simulink model "Projeto_Final_versao_1_M24"  (R2024b)
settings: Solver=VariableStepAuto  StartTime=0  StopTime=144  FixedStep=0.1  RelTol=1e-3
model workspace (MAT data in the model file):
  variavelteste = 0
libraries: visiontextngfix x2, spsACVoltageSourceLib x1, spsCurrentMeasurementLib x1, spsSeriesRLCBranchLib x1, spspowerguiLib x1
settings Model: Creator=Henrique  LastModifiedBy=Guilherme Moreira
settings DebuggingCC: UnconnectedInputMsg=warning  UnconnectedOutputMsg=warning  UnconnectedLineMsg=warning
settings ModelReferenceCC: EnableRefExpFcnMdlSchedulingChecks=on
settings RTWCC: GPUComputeCapability=3.5  DLArmComputeVersion=19.05

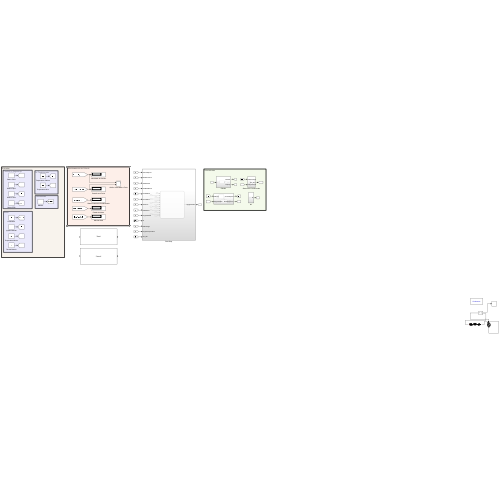
[thumbnail: Simulink's stored preview of the top-level diagram]
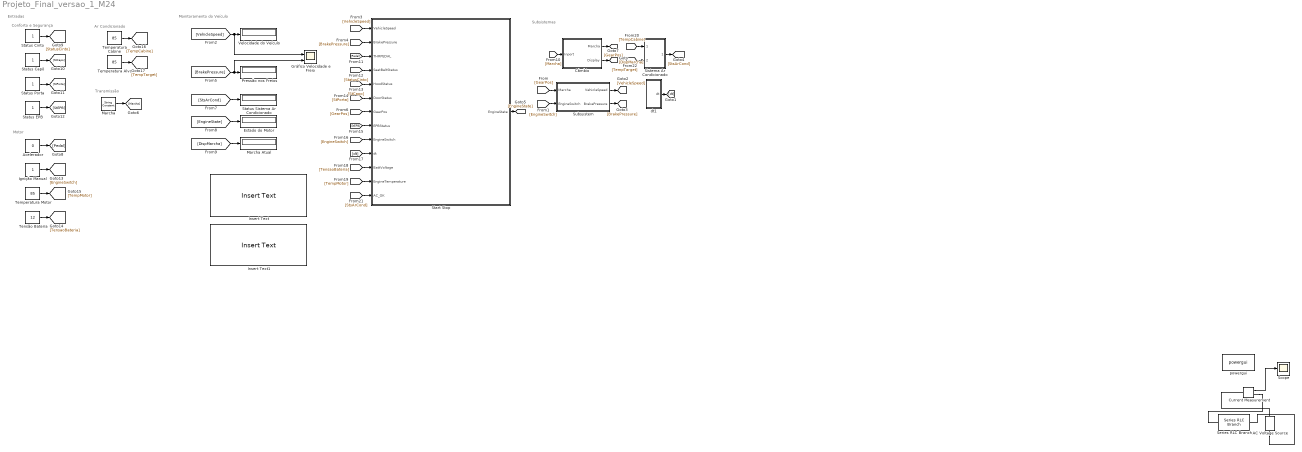
== system Projeto_Final_versao_1_M24 ==
  note: Transmissão
  note: Motor
  note: Conforto e Segurança
  note: Ar Condicionado
  note: Entradas
  note: Subsistemas
  note: Monitoramento do Veículo
  AC Voltage Source : spsACVoltageSourceLib/AC Voltage Source  Amplitude=100  Phase=0  Frequency=60  SampleTime=0  Measurements=None  BusType=swing  Pref=10e3  Qref=0  Qmin=-inf  Qmax=+inf
  Acelerador : Constant  Value=0
  Current Measurement : spsCurrentMeasurementLib/Current Measurement  PhasorSimulation=off  OutputType=Complex  PSBequivalent=0
  Câmbio : Subsystem
  Estado do Motor : Display
  Gráfico Velocidade e Freio : Scope  NumInputPorts=2
  Ignição Manual : Constant
  Insert Text : visiontextngfix/Insert Text  inputType=Obsolete  theText='Teste'  getTextLocFrom=Specify via dialog  textLoc=[1 1]  getTextColorFrom=Specify via dialog  textColor=[0 0 0]  getTextIntensityFrom=Specify via dialog  textIntensity=0  getTextOpacityFrom=Specify via dialog  textOpacity=1.0  dummyVar2=0  dummyVar3=0  dummyVar4=0  imagePorts=One multidimensional signal  isInputTransposed=off  fontFace=LucidaSansRegular  dummyVar1=0  blockFontSize=12  antiAliased=on
  Insert Text1 : visiontextngfix/Insert Text  inputType=Obsolete  theText='Teste2'  getTextLocFrom=Specify via dialog  textLoc=[1 1]  getTextColorFrom=Specify via dialog  textColor=[0 0 0]  getTextIntensityFrom=Specify via dialog  textIntensity=0  getTextOpacityFrom=Specify via dialog  textOpacity=1.0  dummyVar2=0  dummyVar3=0  dummyVar4=0  imagePorts=One multidimensional signal  isInputTransposed=off  fontFace=LucidaSansRegular  dummyVar1=0  blockFontSize=12  antiAliased=on
  Marcha : StringConstant  String="\"D\""
  Marcha Atual : Display
  Pressão nos Freios : Display
  Scope : Scope
  Series RLC Branch : spsSeriesRLCBranchLib/Series RLC Branch  LConnTagsString=__new0  RConnTagsString=__new0  BranchType=RLC  Resistance=1  Inductance=1e-3  SetiL0=off  InitialCurrent=0  Capacitance=1e-6  Setx0=off  InitialVoltage=0  Measurements=None
  Sistema Ar Condicionado : Subsystem
  Start Stop : Subsystem
  Status Capô : Constant
  Status Cinto : Constant
  Status EPB : Constant
  Status Porta : Constant
  Status Sistema Ar Condicionado : Display
  Subsystem : Subsystem
  Temperatura Alvo : Constant  Value=85
  Temperatura Cabine : Constant  Value=85
  Temperatura Motor : Constant  Value=85
  Tensão Bateria : Constant  Value=12
  Velocidade do Veículo : Display
  dt1 : Subsystem
  powergui : spspowerguiLib/powergui  Priority=1  SimulationMode=Continuous  SampleTime=50e-6  frequency=60  Iterations=50  frequencyindice=60  Pbase=100e6  ErrMax=1e-4  UnitsV=kV  UnitsW=MW  buscounter=0  FunctionMessages=off  echomessages=off  EnableUseOfTLC=off  CurrentSourceSwitches=off  DisableSnubberDevices=off  DisableRonSwitches=off  DisableVfSwitches=off  DisplayEquations=off  AutomaticDiscreteSolvers=off  SolverType=Tustin/Backward Euler (TBE)  Interpol=off  ExternalGateDelay=off  methode=off  Ts=100  x0status=blocks  SPID=on  SwTol=0  HookPort=off  NonlinearTolerance=1e-4  nMaxIteration=100  ContinueOnMaxIteration=off  RestoreLinks=warning  ResistiveCurrentMeasurement=off  Frange=[0:2:500]  Ylog=off  Xlog=on  ShowGrid=off  save=off  variable=ZData  structure=0  ZoomFFT=off  StartTime=0.0  cycles=1  DisplayStyle=1  fundamental=60  FreqAxis=off  MaxFrequency=1000  frequencyindicesteady=1  RmsSteady=1  display=off
  wires:
  Current Measurement/1 -> Scope/1
  [dt] -> Start Stop/10(dt)
  Start Stop/1(EngineState) -> [EngineState]
  Sistema Ar Condicionado/1(AC_OK) -> [StsArCond]
  [VehicleSpeed] -> Start Stop/1(VehicleSpeed)
  [BrakePressure] -> Start Stop/2(BrakePressure)
  [VehicleSpeed] -> Gráfico Velocidade e Freio/1, Velocidade do Veículo/1
  [BrakePressure] -> Gráfico Velocidade e Freio/2, Pressão nos Freios/1
  [StsArCond] -> Status Sistema Ar Condicionado/1
  [EngineState] -> Estado do Motor/1
  [DispMarcha] -> Marcha Atual/1
  Marcha/1 -> [Marcha]
  [Marcha] -> Câmbio/1(Inport)
  Câmbio/1(Marcha) -> [GearPos]
  Câmbio/2(Display) -> [DispMarcha]
  [GearPos] -> Start Stop/7(GearPos)
  Acelerador/1 -> [Pedal]
  Status Cinto/1 -> [StatusCinto]
  Status Capô/1 -> [StCapo]
  Status Porta/1 -> [StPorta]
  Status EPB/1 -> [StEPB]
  Ignição Manual/1 -> [EngineSwitch]
  [Pedal] -> Start Stop/3(THRPEDAL)
  [StatusCinto] -> Start Stop/4(SeatBeltStatus)
  [StCapo] -> Start Stop/5(HoodStatus)
  [StPorta] -> Start Stop/6(DoorStatus)
  [StEPB] -> Start Stop/8(EPBStatus)
  [EngineSwitch] -> Start Stop/9(EngineSwitch)
  dt1/1(dt) -> [dt]
  Tensão Bateria/1 -> [TensaoBateria]
  [TensaoBateria] -> Start Stop/11(BattVoltage)
  [TempMotor] -> Start Stop/12(EngineTemperature)
  Temperatura Motor/1 -> [TempMotor]
  [StsArCond] -> Start Stop/13(AC_OK)
  [GearPos] -> Subsystem/1(Marcha)
  [EngineSwitch] -> Subsystem/2(EngineSwitch)
  Subsystem/1(VehicleSpeed) -> [VehicleSpeed]
  Subsystem/2(BrakePressure) -> [BrakePressure]
  Temperatura Alvo/1 -> [TempTarget]
  Temperatura Cabine/1 -> [TempCabine]
  [TempCabine] -> Sistema Ar Condicionado/1(CabinTemperature)
  [TempTarget] -> Sistema Ar Condicionado/2(TargetTemperature)
  connections:
  AC Voltage Source/LConn1 -- Series RLC Branch/RConn1
  AC Voltage Source/RConn1 -- Current Measurement/LConn1
  Current Measurement/RConn1 -- Series RLC Branch/LConn1

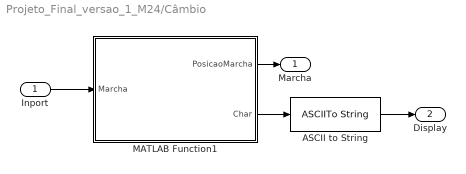
== system Projeto_Final_versao_1_M24/Câmbio ==
  Inport : Inport
  ASCII to String : ASCIIToString
  MATLAB Function1 : MATLAB Function  TreatAsAtomicUnit=on
  Marcha : Outport
  Display : Outport  Port=2
  wires:
  MATLAB Function1/1(PosicaoMarcha) -> Marcha/1
  MATLAB Function1/2(Char) -> ASCII to String/1
  ASCII to String/1 -> Display/1
  Inport/1 -> MATLAB Function1/1(Marcha)

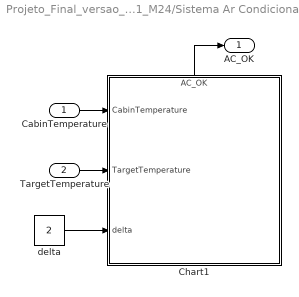
== system Projeto_Final_versao_1_M24/Sistema Ar Condicionado ==
  CabinTemperature : Inport
  TargetTemperature : Inport  Port=2
  Chart1 : Stateflow chart  TreatAsAtomicUnit=on
      settings: PortSchema="{\"entries\":[{\"content\":{\"sides\":[{\"content\":{\"connectorIds\":[\"In1\",\"In2\",\"In3\"]},\"type\":\"ConnectorPlacement.EquallySpacedRectSide\",\"uuid\":\"3dcc586e-91d0-4cd1-aed7-6dda3adf5149\"},{\"content\":{\"side\":\"RIGHT\"},\"type\":\"ConnectorPlacement.EquallySpacedRectSide\",\"uuid\":\"6a827bb4-538e-49ed-9fcc-bcf1675a0976\"},{\"content\":{\"connectorIds\":[\"Out1\"],\"side\":\"TOP\"},\"type\":\"ConnectorPlacement.EquallySpacedRectSide\",\"uuid\":\"8af03e4c-b384-4eb2-b8cc-d6be61dc8da4\"}]},\"type\":\"ConnectorPlacement.EquallySpacedConnector\",\"uuid\":\"bd7ebad6-2738-4989-9528-f935edcb496d\"}],\"packageUris\":[\"http://schema.mathworks.com/mf0/Connector/R2020b\"],\"version\":\"1.0\"}"
  delta : Constant  Value=2
  AC_OK : Outport
  wires:
  Chart1/1(AC_OK) -> AC_OK/1
  delta/1 -> Chart1/3(delta)
  CabinTemperature/1 -> Chart1/1(CabinTemperature)
  TargetTemperature/1 -> Chart1/2(TargetTemperature)

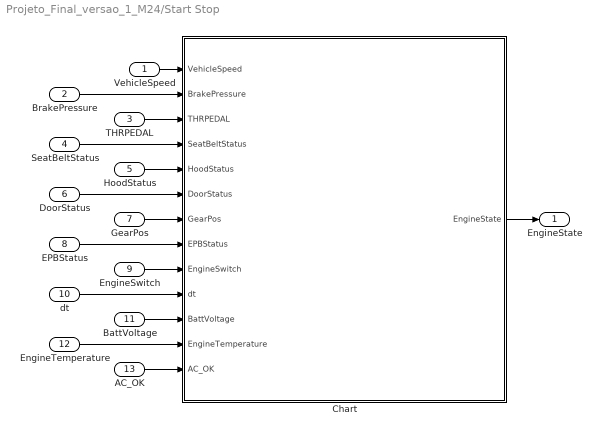
== system Projeto_Final_versao_1_M24/Start Stop ==
  VehicleSpeed : Inport
  BrakePressure : Inport  Port=2
  THRPEDAL : Inport  Port=3
  SeatBeltStatus : Inport  Port=4
  HoodStatus : Inport  Port=5
  DoorStatus : Inport  Port=6
  GearPos : Inport  Port=7
  EPBStatus : Inport  Port=8
  EngineSwitch : Inport  Port=9
  dt : Inport  Port=10
  BattVoltage : Inport  Port=11
  EngineTemperature : Inport  Port=12
  AC_OK : Inport  Port=13
  Chart : Stateflow chart  TreatAsAtomicUnit=on
  EngineState : Outport
  wires:
  Chart/1(EngineState) -> EngineState/1
  THRPEDAL/1 -> Chart/3(THRPEDAL)
  EngineTemperature/1 -> Chart/12(EngineTemperature)
  AC_OK/1 -> Chart/13(AC_OK)
  BattVoltage/1 -> Chart/11(BattVoltage)
  VehicleSpeed/1 -> Chart/1(VehicleSpeed)
  GearPos/1 -> Chart/7(GearPos)
  BrakePressure/1 -> Chart/2(BrakePressure)
  dt/1 -> Chart/10(dt)
  HoodStatus/1 -> Chart/5(HoodStatus)
  DoorStatus/1 -> Chart/6(DoorStatus)
  EngineSwitch/1 -> Chart/9(EngineSwitch)
  EPBStatus/1 -> Chart/8(EPBStatus)
  SeatBeltStatus/1 -> Chart/4(SeatBeltStatus)

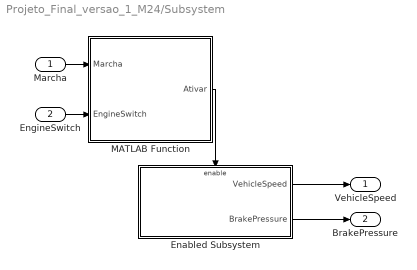
== system Projeto_Final_versao_1_M24/Subsystem ==
  Marcha : Inport
  EngineSwitch : Inport  Port=2
  Enabled Subsystem : Subsystem  TreatAsAtomicUnit=on
  MATLAB Function : MATLAB Function  TreatAsAtomicUnit=on
  VehicleSpeed : Outport
  BrakePressure : Outport  Port=2
  wires:
  Enabled Subsystem/1(VehicleSpeed) -> VehicleSpeed/1
  MATLAB Function/1(Ativar) -> Enabled Subsystem/Enable
  Marcha/1 -> MATLAB Function/1(Marcha)
  Enabled Subsystem/2(BrakePressure) -> BrakePressure/1
  EngineSwitch/1 -> MATLAB Function/2(EngineSwitch)

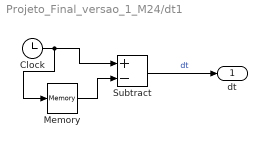
== system Projeto_Final_versao_1_M24/dt1 ==
  Clock : Clock
  Memory : Memory
  Subtract : Sum  Inputs=+-
  dt : Outport
  wires:
  Memory/1 -> Subtract/2
  Clock/1 -> Memory/1, Subtract/1
  Subtract/1 -> dt/1  "dt"

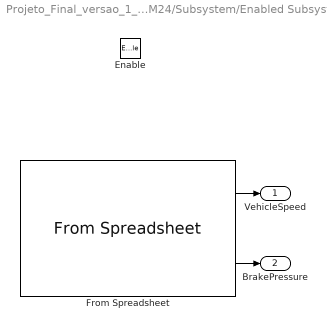
== system Projeto_Final_versao_1_M24/Subsystem/Enabled Subsystem ==
  Enable : EnablePort
  From Spreadsheet : FromSpreadsheet  FileName=tempo.xlsx  SheetName=tempo  Range=A1:C1441  SampleTime=-1
  VehicleSpeed : Outport  InitialOutput=0  VectorParamsAs1DForOutWhenUnconnected=off
  BrakePressure : Outport  Port=2  InitialOutput=0  VectorParamsAs1DForOutWhenUnconnected=off
  wires:
  From Spreadsheet/1 -> VehicleSpeed/1
  From Spreadsheet/2 -> BrakePressure/1

== matlab function Projeto_Final_versao_1_M24/Câmbio/MATLAB Function1 ==
  data: Marcha input; PosicaoMarcha output; Char output
function [PosicaoMarcha,Char] = ConverterMarcha(Marcha)

if Marcha == 'P'
    PosicaoMarcha = 1; 
    Char = uint8(80);
elseif Marcha == 'N'
    PosicaoMarcha = 2; 
    Char = uint8(78);
elseif Marcha == 'D'
    PosicaoMarcha = 3; 
    Char = uint8(68);
elseif Marcha == 'R'
    PosicaoMarcha = 4; 
    Char = uint8(82);
else 
    PosicaoMarcha = 0;
    Char = uint8(69);
end

== stateflow chart Projeto_Final_versao_1_M24/Sistema Ar Condicionado/Chart1 ==
  state AC_Normal
    entry:
    AC_OK = 1;
  state AC_Block
    entry:
    AC_OK = 0;
  (default) -> AC_Normal
  AC_Block -> AC_Normal : [abs(CabinTemperature - TargetTemperature) <= delta]
  AC_Normal -> AC_Block : [abs(CabinTemperature - TargetTemperature) > delta]
  data: CabinTemperature input; TargetTemperature input double; delta input; AC_OK output double

== matlab function Projeto_Final_versao_1_M24/Subsystem/MATLAB Function ==
  data: Marcha input; Ativar output; EngineSwitch input
function Ativar = AtivarSubSistema(Marcha,EngineSwitch)

%A marcha igual a 3 significa que o carro está no "D" - Modo Drive

if ((Marcha==3) && (EngineSwitch==1))  
    Ativar = 1;
else 
    Ativar = 0;
end

== stateflow chart Projeto_Final_versao_1_M24/Start Stop/Chart ==
  state EngineON1
    entry:
    EngineState = 1;  % Motor ligado
    tempo_minimo_ligado = 0;  % Reseta o contador ao entrar no estado
    during:
    tempo_minimo_ligado = tempo_minimo_ligado + dt;  % Incrementa usando dt real da simulação
  state EngineOFF1
    EngineState = 0;  % Motor desligado
  state AutoStop1
    EngineState = 0;  % Motor desligado temporariamente
  EngineON1 -> EngineOFF1 [order 1] : [EngineSwitch == 0
      | ]
  EngineOFF1 -> EngineON1 : [EngineSwitch == 1
      | ]
  AutoStop1 -> EngineON1 : [(BrakePressure < 0.2) || (AC_OK == 0) || (DoorStatus == 0) || (SeatBeltStatus == 0) || (BattVoltage < 12) || (EPBStatus == 1) || (GearPos == 1) || (GearPos == 4)
      | ]
  EngineON1 -> AutoStop1 [order 2] : [((GearPos == 3) || (GearPos == 2)) && (BrakePressure > 0.7) && (VehicleSpeed==0) && (EngineTemperature > 80) && (AC_OK == 1) && (BattVoltage > 12) && (DoorStatus == 1) && (EPBStatus == 0) && (SeatBeltStatus == 1) && (HoodStatus == 1) ]
  (default) -> EngineOFF1
  data: VehicleSpeed input; BrakePressure input; THRPEDAL input; SeatBeltStatus input; HoodStatus input; DoorStatus input; GearPos input; EPBStatus input; EngineState output double; EngineSwitch input double; tempo_minimo_ligado local double =0; dt input =0.01; BattVoltage input; EngineTemperature input; AC_OK input
